simulink model "Week1_problem2"  (R2020b)
settings: Solver=VariableStepAuto  StartTime=0.0  StopTime=10.0  RelTol=1e-3
model workspace (MAT data in the model file):
  M1 = 0.01
  M2 = 0.5
  b = 50
  k1 = 50
  k2 = 1
  out = Simulink.SimulationOutput
  out.Data.tout = [0 0.0002 0.0004 0.0006 0.0008 0.001 0.0012 0.0014 0.0016 0.0018 0.002 0.0022 ... (50001 elements, 50001x1)]
  out.Metadata = Simulink.SimulationMetadata
  out.Metadata.ModelInfo.ModelName = 'week1_problem1'
  out.Metadata.ModelInfo.ModelVersion = '1.7'
  out.Metadata.ModelInfo.ModelFilePath = 'E:\MY MATLAB PROJECT\Week1_Problem1\Model\week1_problem1.slx'
  out.Metadata.ModelInfo.UserID = 'sai'
  out.Metadata.ModelInfo.MachineName = 'DESKTOP-L87NR0P'
  out.Metadata.ModelInfo.Platform = 'PCWIN64'
  out.Metadata.ModelInfo.ModelStructuralChecksum = [3684594609; 3024041146; 535422527; 4070629996]
  out.Metadata.ModelInfo.SimulationMode = 'normal'
  out.Metadata.ModelInfo.StartTime = 0
  out.Metadata.ModelInfo.StopTime = 10
  out.Metadata.ModelInfo.SolverInfo.Type = 'Variable-Step'
  out.Metadata.ModelInfo.SolverInfo.Solver = 'ode45'
  out.Metadata.ModelInfo.SolverInfo.MaxStepSize = 0.0002
  out.Metadata.ModelInfo.SimulinkVersion.Name = 'Simulink'
  out.Metadata.ModelInfo.SimulinkVersion.Version = '10.2'
  out.Metadata.ModelInfo.SimulinkVersion.Release = '(R2020b)'
  out.Metadata.ModelInfo.SimulinkVersion.Date = '29-Jul-2020'
  out.Metadata.ModelInfo.LoggingInfo.LoggingToFile = 'off'
  out.Metadata.TimingInfo.WallClockTimestampStart = '2021-03-11 03:12:40'
  out.Metadata.TimingInfo.WallClockTimestampStop = '2021-03-11 03:12:44'
  out.Metadata.TimingInfo.InitializationElapsedWallTime = 2.618162539
  out.Metadata.TimingInfo.ExecutionElapsedWallTime = 1.038026164
  out.Metadata.TimingInfo.TerminationElapsedWallTime = 0.04913768
  out.Metadata.TimingInfo.TotalElapsedWallTime = 3.705326383
  out.Metadata.TimingInfo.ProfilerData = 'Profiler is not enabled'
  out.Metadata.ExecutionInfo.StopEvent = 'ReachedStopTime'
  out.Metadata.ExecutionInfo.StopEventSource = []
  out.Metadata.ExecutionInfo.StopEventDescription = 'Reached stop time of 10'
  out.Metadata.ExecutionInfo.ErrorDiagnostic = []
  out.Metadata.ExecutionInfo.WarningDiagnostics = struct([])
  out.Metadata.AppInfo = struct()
settings Model: Creator=sai  LastModifiedBy=sai

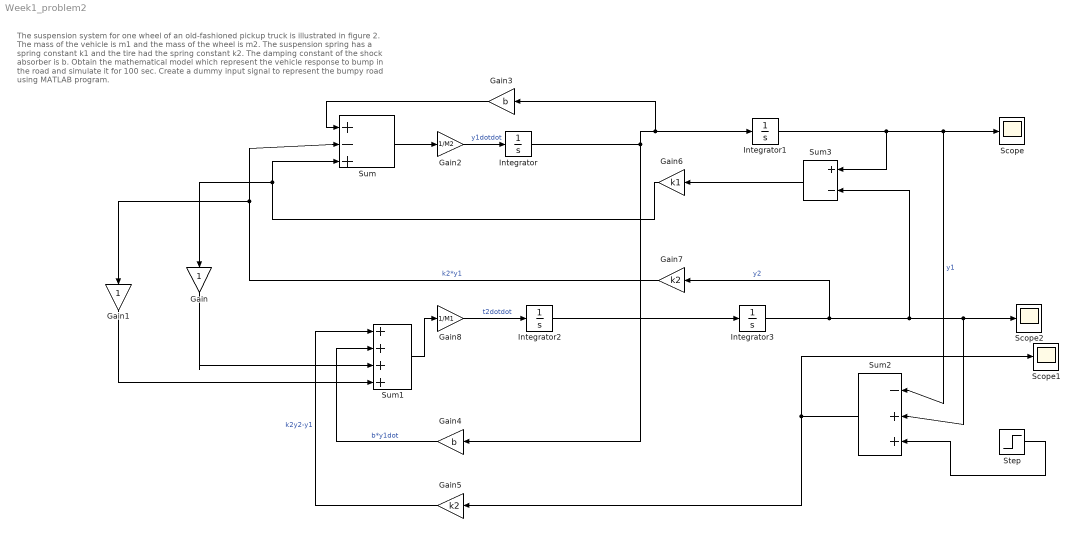
== system Week1_problem2 ==
  note: The suspension system for one wheel of an old-fashioned pickup truck is illustrated in figure 2. The mass of the vehicle is m1 and the mass of the wheel is m2. The suspension spring has a spring constant k1 and the tire had the spring constant k2. The damping constant of the shock absorber is b. Obtain the mathematical model which represent the vehicle response to bump in the road and simulate it for 100 sec. Create a dummy input signal to represent the bumpy road using MATLAB program.
  Gain : Gain
  Gain1 : Gain
  Gain2 : Gain  Gain=1/M2
  Gain3 : Gain  Gain=b
  Gain4 : Gain  Gain=b
  Gain5 : Gain  Gain=k2
  Gain6 : Gain  Gain=k1
  Gain7 : Gain  Gain=k2
  Gain8 : Gain  Gain=1/M1
  Integrator{,1..3} (4 alike) : Integrator
  Scope : Scope
  Scope1 : Scope
  Scope2 : Scope
  Step : Step  SampleTime=0
  Sum : Sum  Inputs=|+-+
  Sum1 : Sum  Inputs=|++++
  Sum2 : Sum  Inputs=|-++
  Sum3 : Sum  Inputs=+-
  wires:
  Gain6/1 -> Sum/3, Gain/1
  Integrator3/1 -> Gain7/1, Sum3/2, Sum2/2, Scope2/1  "y2"
  Gain2/1 -> Integrator/1  "y1dotdot"
  Integrator/1 -> Integrator1/1, Gain3/1, Gain4/1
  Step/1 -> Sum2/3
  Integrator1/1 -> Sum2/1, Scope/1, Sum3/1  "y1"
  Sum1/1 -> Gain8/1
  Sum3/1 -> Gain6/1
  Gain4/1 -> Sum1/2  "b*y1dot"
  Sum2/1 -> Gain5/1, Scope1/1
  Gain5/1 -> Sum1/1  "k2y2-y1"
  Gain/1 -> Sum1/3
  Integrator2/1 -> Integrator3/1
  Gain3/1 -> Sum/1
  Gain7/1 -> Gain1/1, Sum/2  "k2*y1"
  Gain1/1 -> Sum1/4
  Gain8/1 -> Integrator2/1  "t2dotdot"
  Sum/1 -> Gain2/1
